simulink model "non_augmented_system"  (R2018b)
settings: Solver=VariableStepAuto  StartTime=0.0  StopTime=10.0  RelTol=1e-3
values from neighbouring files (symbols this model uses):
  Am = [-0.5 0 0 0 0 0 0 0 ... (first row only)    [Dynamic_model_articulation.m]
  Bm = [1;0;0;0]    [Dynamic_model_articulation.m]
  Bp = B2    [Dynamic_model_articulation.m]    (also in articulation.m = M_inv*delta)
  constants = [C1 C2 C3 m1 m2 I1 I2 a1 l1 h1 b1 a2 l2 Vx]    [Dynamic_model_articulation.m]
  N2 = 2    [Dynamic_model_articulation.m]
  Pm = lyap(Am,Q)    [Dynamic_model_articulation.m]
settings Model: Creator=kevingasik  LastModifiedBy=kevingasik

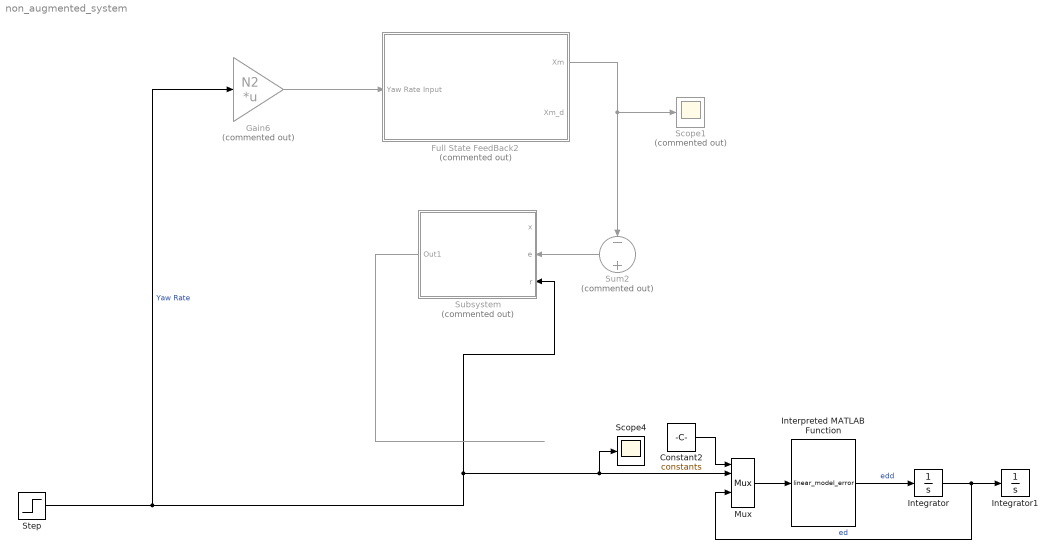
== system non_augmented_system ==
  Constant2 : Constant  Value=constants
  Full State FeedBack2 : Subsystem  Commented=on
  Gain6 : Gain  Commented=on  Gain=N2  Multiplication=Matrix(K*u)
  Integrator : Integrator
  Integrator1 : Integrator
  Interpreted MATLAB Function : MATLABFcn  MATLABFcn=linear_model_error  OutputDimensions=4
  Mux : Mux  Inputs=5
  Scope1 : Scope  Commented=on
  Scope4 : Scope
  Step : Step  Time=0  After=0.5*pi/180  SampleTime=0
  Subsystem : Subsystem  Commented=on
  Sum2 : Sum  Commented=on  Inputs=-+
  wires:
  Interpreted MATLAB Function/1 -> Integrator/1  "edd"
  Gain6/1 -> Full State FeedBack2/1(Yaw Rate Input)
  Full State FeedBack2/1(Xm) -> Sum2/1, Scope1/1
  Sum2/1 -> Subsystem/2(e)
  Constant2/1 -> Mux/1
  Step/1 -> Mux/2, Scope4/1, Subsystem/3(r), Gain6/1  "Yaw Rate"
  Mux/1 -> Interpreted MATLAB Function/1
  Subsystem/1(Out1) -> ?
  Integrator/1 -> Mux/4, Integrator1/1  "ed"
  ? -> Mux/3

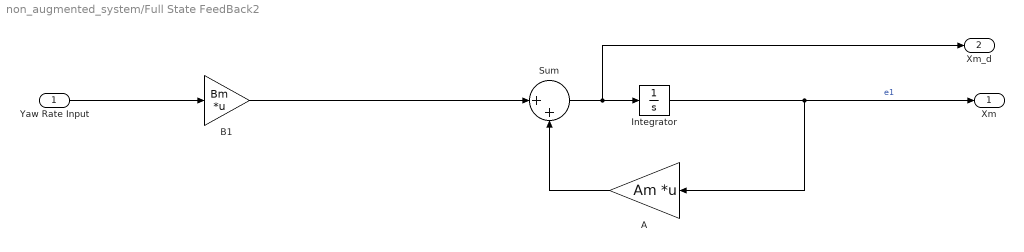
== system non_augmented_system/Full State FeedBack2 ==
  Yaw Rate Input : Inport
  A : Gain  Gain=Am  Multiplication=Matrix(K*u)
  B1 : Gain  Gain=Bm  Multiplication=Matrix(K*u)
  Integrator : Integrator
  Sum : Sum  Inputs=|++
  Xm : Outport
  Xm_d : Outport  Port=2
  wires:
  Sum/1 -> Xm_d/1, Integrator/1
  A/1 -> Sum/2
  Integrator/1 -> Xm/1, A/1  "e1"
  Yaw Rate Input/1 -> B1/1
  B1/1 -> Sum/1

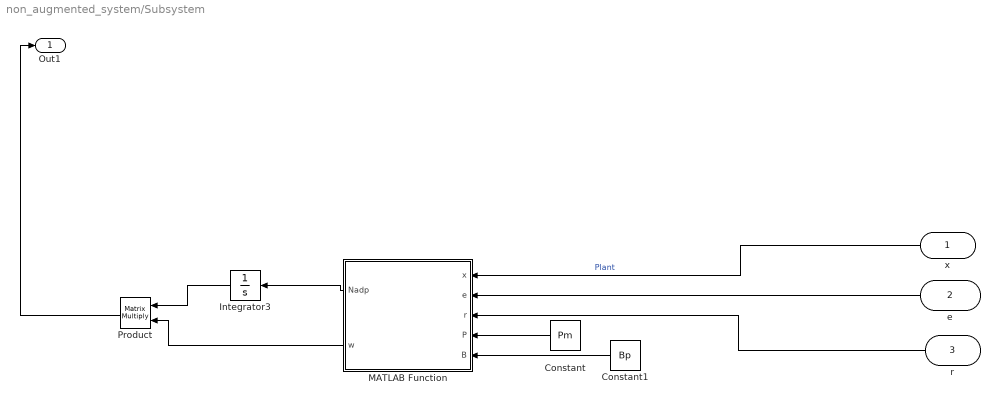
== system non_augmented_system/Subsystem ==
  x : Inport
  e : Inport  Port=2
  r : Inport  Port=3
  Constant : Constant  Value=Pm  VectorParams1D=off
  Constant1 : Constant  Value=Bp  VectorParams1D=off
  Integrator3 : Integrator
  MATLAB Function : MATLAB Function  TreatAsAtomicUnit=on
  Product : Product  Multiplication=Matrix(*)
  Out1 : Outport
  wires:
  r/1 -> MATLAB Function/3(r)
  MATLAB Function/2(w) -> Product/2
  Constant/1 -> MATLAB Function/4(P)
  x/1 -> MATLAB Function/1(x)  "Plant"
  Integrator3/1 -> Product/1
  Product/1 -> Out1/1
  MATLAB Function/1(Nadp) -> Integrator3/1
  e/1 -> MATLAB Function/2(e)
  Constant1/1 -> MATLAB Function/5(B)

== matlab function non_augmented_system/Subsystem/MATLAB Function ==
  data: x input; Nadp output; e input; r input; P input; w output; B input
function [Nadp,w]   = fcn(x,e,r,P,B)

w = [0;0;0;0;0;0];
Nadp = [0;0;0;0;0;0]';

%x = [0; x(2);x(3);x(4)];
%e = [0; e(2);e(3);e(4)];

%x = [x(1);0;0;0];
%e = [e(1);0;0;0];


%% define learning rate
gr = 0.5; 
gx = [1 0 0 0;
      0 1 0 0;
      0 0 1 0;
      0 0 0 1];

ydd = 0.5;

%% Thesis paper
w = [x' r 1]';
 
theta_xd = -gx*x*e'*P*B;
theta_d_d = -ydd*e'*P*B;
theta_rd = -gr*e'*P*B;

Nadp = [theta_xd' theta_d_d' theta_rd']
